simulink model "matematisk_modell_av_dc_motor"  (R2023a)
settings: Solver=VariableStepAuto  StartTime=0.0  StopTime=50  RelTol=1e-3
values from neighbouring files (symbols this model uses):
  b = J/Tau_m    (= 7.93103448276e-05)    [matematisk_model_parametere.m]
  J = 25.3*10^-7    (= 2.53e-06)    [matematisk_model_parametere.m]
  Kb = (1/344)*((2*pi)/60)    (= 0.00030441789279)    [matematisk_model_parametere.m]
  Kt = 27.8*10^-3    (= 0.0278)    [matematisk_model_parametere.m]
  L = 1.27*10^-3    (= 0.00127)    [matematisk_model_parametere.m]
  R = 9.73    [matematisk_model_parametere.m]
  TL = 0    [matematisk_model_parametere.m]
settings Model: Creator=mahna  LastModifiedBy=mahna

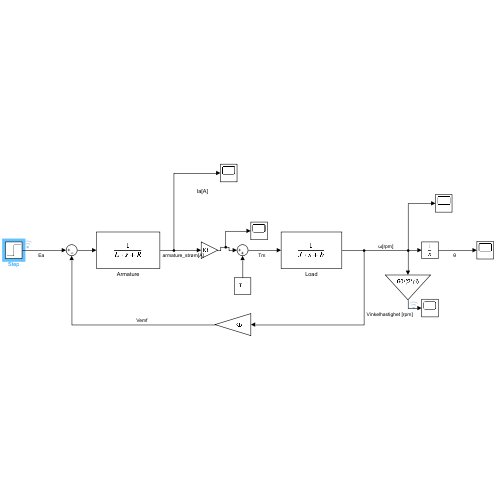
[thumbnail: Simulink's stored preview of the top-level diagram]
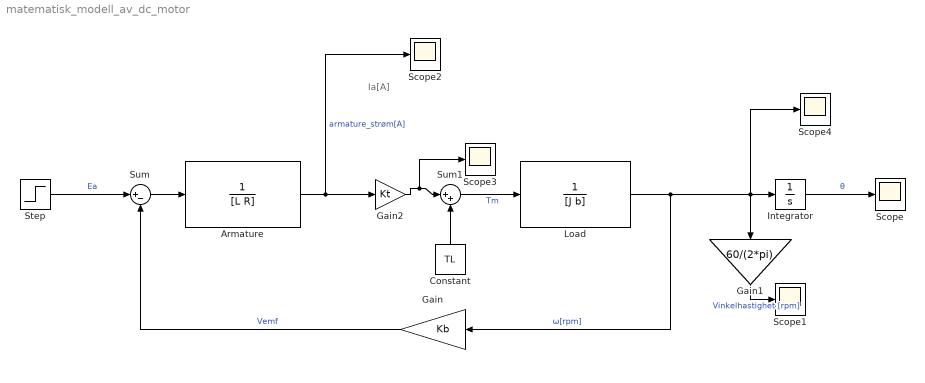
== system matematisk_modell_av_dc_motor ==
  note: Ia[A]
  Armature : TransferFcn  Denominator=[L R]
  Constant : Constant  Value=TL
  Gain : Gain  Gain=Kb
  Gain1 : Gain  Gain=60/(2*pi)
  Gain2 : Gain  Gain=Kt
  Integrator : Integrator
  Load : TransferFcn  Denominator=[J b]
  Scope{,1..4} (5 alike) : Scope
  Step : Step  Time=0  After=2.54  SampleTime=0
  Sum : Sum  Inputs=|+-
  Sum1 : Sum  Inputs=|++
  wires:
  Sum/1 -> Armature/1
  Load/1 -> Gain/1, Gain1/1, Scope4/1, Integrator/1  "ω[rpm]"
  Gain/1 -> Sum/2  "Vemf"
  Step/1 -> Sum/1  "Ea"
  Constant/1 -> Sum1/2
  Sum1/1 -> Load/1  "Tm"
  Integrator/1 -> Scope/1  "θ"
  Gain1/1 -> Scope1/1  "Vinkelhastighet [rpm]"
  Armature/1 -> Scope2/1, Gain2/1  "armature_strøm[A]"
  Gain2/1 -> Scope3/1, Sum1/1
